simulink model "sldemo_mdlref_counter"  (R2021a)
settings: Solver=FixedStepDiscrete  StartTime=0.0  StopTime=10.0  FixedStep=Auto  RelTol=1e-3  EnableMultiTasking=on
settings Model: ModifiedByFormat=The MathWorks Inc.  ExtModeAutoUpdateStatusClock=off  Creator=The MathWorks, Inc.  LastModifiedBy=The MathWorks Inc.
settings SolverCC: AlgebraicLoopSolver=TrustRegion
settings DataIOCC: LimitDataPoints=on  SaveFinalState=on  SaveState=on  SignalLoggingName=logsOut
settings OptimizationCC: DefaultParameterBehavior=Inlined  InlineInvariantSignals=on  ExpressionDepthLimit=2147483647  InitFltsAndDblsToZero=on  LifeSpan=inf
settings DebuggingCC: SaveWithParameterizedLinksMsg=none  CheckExecutionContextPreStartOutputMsg=on  MultiTaskDSMMsg=warning  MultiTaskCondExecSysMsg=none  SigSpecEnsureSampleTimeMsg=none  FcnCallInpInsideContextMsg=warning  AllowSymbolicDim=off  StateNameClashWarn=warning  StrictBusMsg=ErrorOnBusTreatedAsVector  SFUnexpectedBacktrackingDiag=warning  SFNoUnconditionalDefaultTransitionDiag=warning  SFExecutionAtInitializationDiag=none  SFMachineParentedDataDiag=warning  ArithmeticOperatorsInVariantConditions=warning
settings HardwareCC: ProdBitPerPointer=32  ProdBitPerSizeT=32  ProdBitPerPtrDiffT=32  ProdLargestAtomicFloat=None  ProdIntDivRoundTo=Undefined  ProdEndianess=Unspecified  ProdWordSize=32  ProdHWDeviceType=32-bit Generic  TargetHWDeviceType=32-bit Generic
settings ModelReferenceCC: UpdateModelReferenceTargets=IfOutOfDate  CheckModelReferenceTargetMessage=none  PropagateSignalLabelsOutOfModel=off
settings SFSimCC: SimUseLocalCustomCode=off  CustomCodeUndefinedFunction=UseInterfaceOnly
settings RTWCC: Description=Generic Real-Time Target  GenerateReport=on  RTWUseLocalCustomCode=off  LaunchReport=on
settings CodeAppCC: MaxIdLength=100  StateflowObjectComments=on
settings GRTTargetCC: TargetFcnLib=ansi_tfl_tmw.mat  TargetLangStandard=C89/C90 (ANSI)  CombineOutputUpdateFcns=off  GRTInterface=on
settings ConfigComp: CovMetricSettings=dw  CovSaveCumulativeToWorkspaceVar=on  CovSaveSingleToWorkspaceVar=on  CovExternalEMLEnable=off  CovSFcnEnable=off

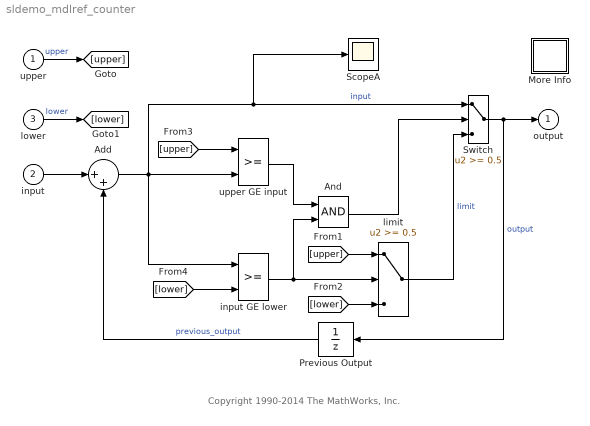
== system sldemo_mdlref_counter ==
  note: Copyright 1990-2014 The MathWorks, Inc.
  " upper" : Inport  OutDataTypeStr=double  PortDimensions=1
  " input" : Inport  Port=2  OutDataTypeStr=double  PortDimensions=1
  lower : Inport  Port=3  OutDataTypeStr=double  PortDimensions=1
  " input GE lower" : RelationalOperator  Priority=1  RndMeth=Nearest  InputSameDT=on
      settings: AttributesFormatString=\n
  " limit" : Switch  Threshold=0.5  SaturateOnIntegerOverflow=on  InputSameDT=on
  Add : Sum  Inputs=|++
  And : Logic
  More Info : Subsystem
      settings: OpenFcn=showExample('simulink_features/ComponentBasedModelingWithModelReferenceExample')
      mask Display: disp('?')
  Previous Output : UnitDelay  SampleTime=-1  HasFrameUpgradeWarning=on
  ScopeA : Scope
  Switch : Switch  Threshold=0.5  SaturateOnIntegerOverflow=on  InputSameDT=on
  upper GE input : RelationalOperator  Priority=0  RndMeth=Nearest  InputSameDT=on
      settings: AttributesFormatString=\n
  output : Outport  VectorParamsAs1DForOutWhenUnconnected=off
  wires:
  [upper] -> " limit"/1
  Switch/1 -> output/1, Previous Output/1  "output"
  " limit"/1 -> Switch/3  "limit"
  upper GE input/1 -> And/1
  Previous Output/1 -> Add/2  "previous_output"
  " input"/1 -> Add/1
  " upper"/1 -> [upper]  "upper"
  [lower] -> " limit"/3
  [upper] -> upper GE input/1
  [lower] -> " input GE lower"/2
  " input GE lower"/1 -> And/2, " limit"/2
  lower/1 -> [lower]  "lower"
  And/1 -> Switch/2
  Add/1 -> upper GE input/2, " input GE lower"/1, Switch/1, ScopeA/1  "input"

== system sldemo_mdlref_counter/More Info ==
  note: Bus Block Demonstration
  note: This demonstration shows how signals may be grouped and ungrouped while
      | retaining their names.  In this demonstration, 5 signals are created and labelled
      | appropriately.  These signals are then mux'd together to create a bus of signals.
      | This bus of signals is then fed into the Bus Selector block.  Inside of the Bus
      | Selector block, the Pulse and Chirp signals are chosen to be output from the
      | original signal bus.
      |
      | It is possible to place a nest signal buses and then still retrieve the original signal
      | with its label.
